simulink model "Assignment1"  (R2020a)
settings: Solver=FixedStepAuto  StartTime=0.0  StopTime=10.0  FixedStep=1e-3  RelTol=1e-3  EnableMultiTasking=on
settings Model: ExtModeTrigDuration=5  Creator=John  LastModifiedBy=John
settings OptimizationCC: EnhancedBackFolding=on  PassReuseOutputArgsAs=Individual arguments  ZeroExternalMemoryAtStartup=off  ZeroInternalMemoryAtStartup=off  MaxStackSize=64  OptimizeBlockOrder=speed  DifferentSizesBufferReuse=on  OptimizationCustomize=off  EfficientTunableParamExpr=on
settings DebuggingCC: ParameterTunabilityLossMsg=error
settings HardwareCC: ProdBitPerPointer=32  ProdBitPerSizeT=32  ProdBitPerPtrDiffT=32  ProdLargestAtomicInteger=Long  ProdLargestAtomicFloat=Double  ProdWordSize=32  ProdHWDeviceType=ARM Compatible->ARM Cortex
settings SFSimCC: MATLABDynamicMemAlloc=off
settings RTWCC: SystemTargetFile=ert.tlc  HardwareBoard=NXP FRDM-K64F  TemplateMakefile=ert_default_tmf  Toolchain=GNU Tools for ARM Embedded Processors
settings CodeAppCC: ForceParamTrailComments=on  IgnoreCustomStorageClasses=off  OperatorAnnotations=on  SimulinkDataObjDesc=on  SFDataObjDesc=on  InsertBlockDesc=on

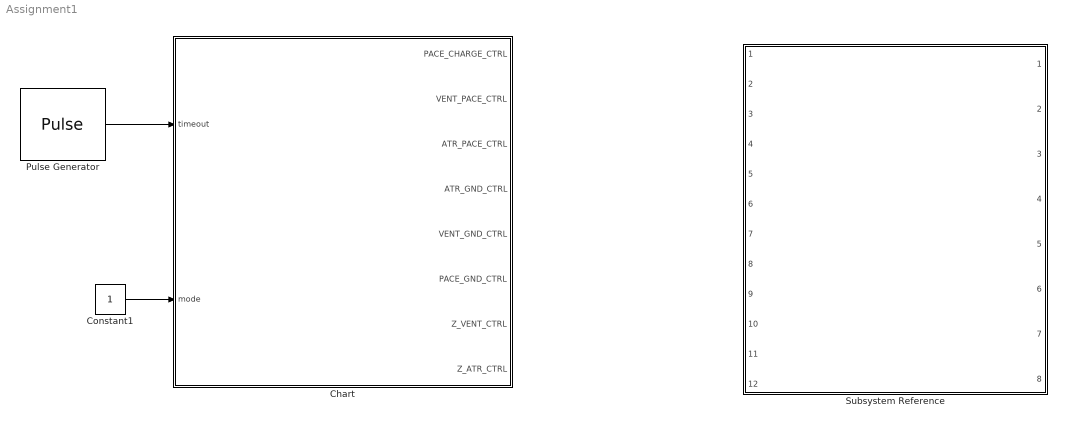
== system Assignment1 ==
  Chart : Stateflow chart  TreatAsAtomicUnit=on
  Constant1 : Constant
  Pulse Generator : DiscretePulseGenerator  PulseType=Time based  Period=1  PulseWidth=50
  Subsystem Reference : Subsystem  ReferencedSubsystem=k64f_subsystem
  wires:
  Pulse Generator/1 -> Chart/1(timeout)
  Constant1/1 -> Chart/2(mode)

== stateflow chart Assignment1/Chart ==
  state CHARGING
    entry:
    PACE_CHARGE_CTRL = 1
  state IDLE
    entry:
    ATR_PACE_CTRL = 0
    VENT_PACE_CTRL = 0
    Z_VENT_CTRL = 1;
    Z_ATR_CTRL = 1;
  state DELAY
  state Select_mode
    entry:
    VENT_GND_CTRL = 0
    ATR_GND_CTRL = 0
  state Atrial_Pacing
    entry:
    ATR_PACE_CTRL = 1
    VENT_PACE_CTRL = 0
    PACE_GND_CTRL = 1;
    Z_VENT_CTRL = 0;
    Z_ATR_CTRL = 0;
  state No_Pacing
    entry:
    ATR_PACE_CTRL = 0
    VENT_PACE_CTRL = 0
  state Ventricular_Pacing
    entry:
    ATR_PACE_CTRL = 0
    VENT_PACE_CTRL = 1
    PACE_GND_CTRL = 1;
    Z_VENT_CTRL = 0;
    Z_ATR_CTRL = 0;
  state Discharging
    entry:
    VENT_GND_CTRL = 1
    ATR_GND_CTRL = 1
  (default) -> IDLE
  Discharging -> IDLE
  IDLE -> CHARGING
  CHARGING -> DELAY
  DELAY -> Select_mode : [timeout == 1]
  Select_mode -> Atrial_Pacing [order 1] : [mode == 1]
  Select_mode -> Ventricular_Pacing [order 2] : [mode == 2]
  Select_mode -> No_Pacing [order 3] : [mode == 3]
  No_Pacing -> Discharging
  Atrial_Pacing -> Discharging
  Ventricular_Pacing -> Discharging
  data: PACE_CHARGE_CTRL output; VENT_PACE_CTRL output; ATR_PACE_CTRL output; timeout input; ATR_GND_CTRL output; VENT_GND_CTRL output; PACE_GND_CTRL output; mode input; Z_VENT_CTRL output; Z_ATR_CTRL output
